simulink model "NL_PID_3fal_MODEL"  (Simulink 7.6)
settings: Solver=ode45  StartTime=0.0  StopTime=20  RelTol=1e-3
settings Model: Creator=Administrator  LastModifiedBy=Administrator
settings DebuggingCC: SolverPrmCheckMsg=none

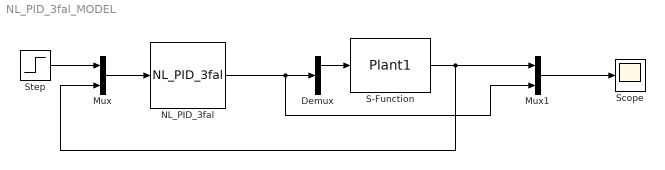
== system NL_PID_3fal_MODEL ==
  Demux : Demux  Outputs=2
  Mux : Mux  Inputs=2
  Mux1 : Mux  Inputs=2
  NL_PID_3fal : S-Function  FunctionName=NL_PID_3fal  Parameters=r0,h0,r1,h1,h,Bet,A,D  EnableBusSupport=off  mask{r0=0.5, h0=0.02, r1=50, h1=0.01, h=0.01, Bet=[30,80,50], A=[0.25,0.75,1.5], D=0.6}
      mask prompts: r0 "r0="; h0 "h0="; r1 "r1="; Bet "Bet="; A "A=[]"; D "D="
  S-Function : S-Function  FunctionName=Plant1  EnableBusSupport=off
  Scope : Scope
      settings: YMin=-11  YMax=3
  Step : Step  Time=0  After=1.5  SampleTime=0
  wires:
  Step/1 -> Mux/1
  Mux/1 -> NL_PID_3fal/1
  Mux1/1 -> Scope/1
  NL_PID_3fal/1 -> Demux/1, Mux1/2
  Demux/1 -> S-Function/1
  S-Function/1 -> Mux1/1, Mux/2
